simulink model "sschdlexNPCBridgeExample"  (R2023b)
settings: Solver=FixedStepDiscrete  StartTime=0.0  StopTime=0.0333  RelTol=1e-3
InitFcn:
  | ts = 1e-6;
libraries: fl_lib x17, nesl_utility x14, ee_lib x4, simulink x2, powerlib_meascontrol x2
CloseFcn:
  | clear all;
settings Model: DataTypeOverride=Off  Creator=The MathWorks, Inc.  LastModifiedBy=The MathWorks, Inc.
settings SolverCC: AlgebraicLoopSolver=TrustRegion
settings OptimizationCC: BlockReduction=off  ConditionallyExecuteInputs=off  DefaultParameterBehavior=Inlined
settings DebuggingCC: AlgebraicLoopMsg=error  SingleTaskRateTransMsg=error  UnconnectedInputMsg=warning  UnconnectedOutputMsg=warning  UnconnectedLineMsg=warning
settings HardwareCC: ProdBitPerPointer=32  ProdBitPerSizeT=32  ProdBitPerPtrDiffT=32  ProdLargestAtomicFloat=None  ProdIntDivRoundTo=Undefined  ProdEndianess=Unspecified  ProdWordSize=32  ProdHWDeviceType=ASIC/FPGA->ASIC/FPGA  TargetBitPerPointer=64  TargetBitPerSizeT=64  TargetBitPerPtrDiffT=64  TargetLongLongMode=on  TargetIntDivRoundTo=Zero  TargetEndianess=LittleEndian  TargetWordSize=64  TargetHWDeviceType=Custom Processor->MATLAB Host Computer  ProdEqTarget=off
settings ModelReferenceCC: EnableRefExpFcnMdlSchedulingChecks=on
settings RTWCC: DLArmComputeVersion=19.05

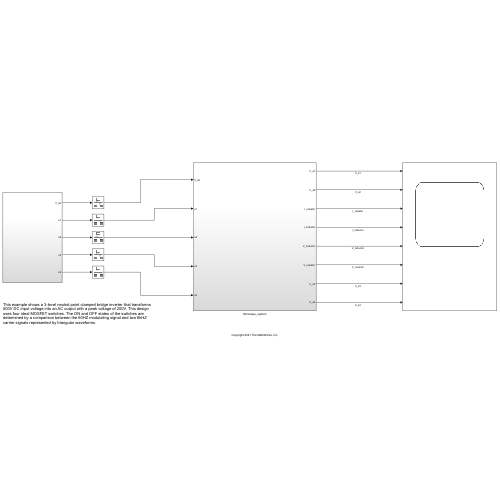
[thumbnail: Simulink's stored preview of the top-level diagram]
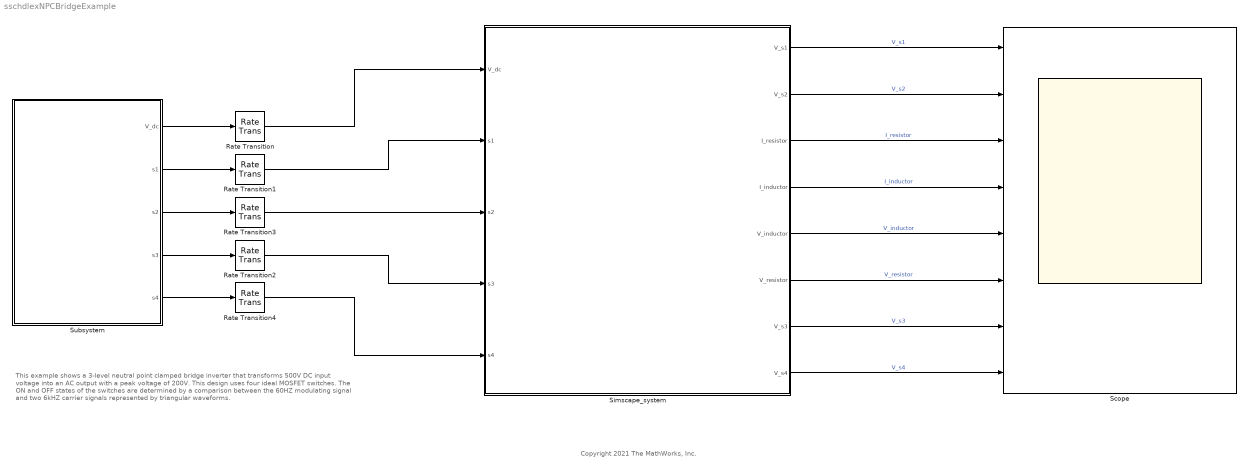
== system sschdlexNPCBridgeExample ==
  note: This example shows a 3-level neutral point clamped bridge inverter that transforms 500V DC input voltage into an AC output with a peak voltage of 200V. This design uses four ideal MOSFET switches. The ON and OFF states of the switches are determined by a comparison between the 60HZ modulating signal and two 6kHZ carrier signals represented by triangular waveforms.
  note: Copyright 2021 The MathWorks, Inc.
  Rate Transition{,1..4} (5 alike) : RateTransition
  Scope : Scope  NumInputPorts=8
  Simscape_system : Subsystem
  Subsystem : Subsystem
  wires:
  Subsystem/5(s4) -> Rate Transition4/1
  Subsystem/3(s2) -> Rate Transition3/1
  Subsystem/4(s3) -> Rate Transition2/1
  Subsystem/2(s1) -> Rate Transition1/1
  Subsystem/1(V_dc) -> Rate Transition/1
  Rate Transition/1 -> Simscape_system/1(V_dc)
  Rate Transition1/1 -> Simscape_system/2(s1)
  Rate Transition3/1 -> Simscape_system/3(s2)
  Rate Transition2/1 -> Simscape_system/4(s3)
  Rate Transition4/1 -> Simscape_system/5(s4)
  Simscape_system/1(V_s1) -> Scope/1  "V_s1"
  Simscape_system/2(V_s2) -> Scope/2  "V_s2"
  Simscape_system/3(I_resistor) -> Scope/3  "I_resistor"
  Simscape_system/4(I_inductor) -> Scope/4  "I_inductor"
  Simscape_system/5(V_inductor) -> Scope/5  "V_inductor"
  Simscape_system/6(V_resistor) -> Scope/6  "V_resistor"
  Simscape_system/7(V_s3) -> Scope/7  "V_s3"
  Simscape_system/8(V_s4) -> Scope/8  "V_s4"

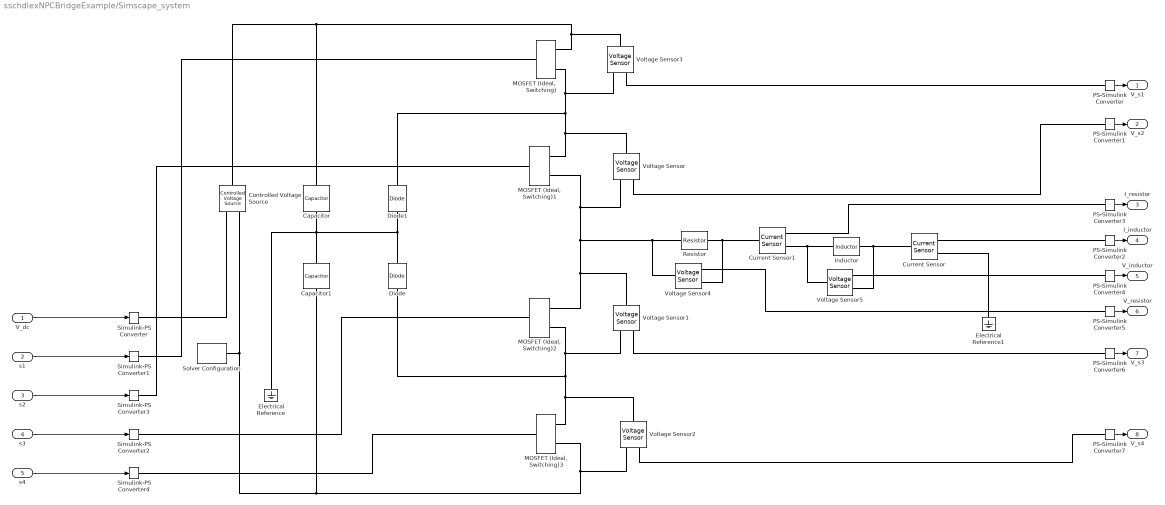
== system sschdlexNPCBridgeExample/Simscape_system ==
  V_dc : Inport
  s1 : Inport  Port=2
  s2 : Inport  Port=3
  s3 : Inport  Port=4
  s4 : Inport  Port=5
  Capacitor : fl_lib/Electrical/Electrical Elements/Capacitor  c=500e-6 F  r=0 Ohm  g=0 1/Ohm  i_specify=off  i_priority=None  i=0 A  i_nominal_specify=off  i_nominal_unit=A  i_nominal_value=1  v_specify=off  v_priority=None  v=250 V  v_nominal_specify=off  v_nominal_unit=V  v_nominal_value=1  vc_specify=on  vc_priority=High  vc=250 V  vc_nominal_specify=off  vc_nominal_unit=V  vc_nominal_value=1
  Capacitor1 : fl_lib/Electrical/Electrical Elements/Capacitor  c=500e-6 F  r=0 Ohm  g=0 1/Ohm  i_specify=off  i_priority=None  i=0 A  i_nominal_specify=off  i_nominal_unit=A  i_nominal_value=1  v_specify=off  v_priority=None  v=250 V  v_nominal_specify=off  v_nominal_unit=V  v_nominal_value=1  vc_specify=on  vc_priority=High  vc=250 V  vc_nominal_specify=off  vc_nominal_unit=V  vc_nominal_value=1
  Controlled Voltage Source : fl_lib/Electrical/Electrical Sources/Controlled Voltage Source
  Current Sensor : fl_lib/Electrical/Electrical Sensors/Current Sensor
  Current Sensor1 : fl_lib/Electrical/Electrical Sensors/Current Sensor
  Diode : fl_lib/Electrical/Electrical Elements/Diode  Vf=0.6 V  Ron=1e-3 Ohm  Goff=1e-8 1/Ohm  i_specify=off  i_priority=None  i=0 A  i_nominal_specify=off  i_nominal_unit=A  i_nominal_value=1  v_specify=off  v_priority=None  v=0 V  v_nominal_specify=off  v_nominal_unit=V  v_nominal_value=1
  Diode1 : fl_lib/Electrical/Electrical Elements/Diode  Vf=0.6 V  Ron=1e-3 Ohm  Goff=1e-8 1/Ohm  i_specify=off  i_priority=None  i=0 A  i_nominal_specify=off  i_nominal_unit=A  i_nominal_value=1  v_specify=off  v_priority=None  v=0 V  v_nominal_specify=off  v_nominal_unit=V  v_nominal_value=1
  Electrical Reference : fl_lib/Electrical/Electrical Elements/Electrical Reference
  Electrical Reference1 : fl_lib/Electrical/Electrical Elements/Electrical Reference
  Inductor : fl_lib/Electrical/Electrical Elements/Inductor  l=200e-3 H  r=0 Ohm  g=1e-9 1/Ohm  i_specify=off  i_priority=None  i=0 A  i_nominal_specify=off  i_nominal_unit=A  i_nominal_value=1  v_specify=off  v_priority=None  v=0 V  v_nominal_specify=off  v_nominal_unit=V  v_nominal_value=1  i_L_specify=off  i_L_priority=High  i_L=0 A  i_L_nominal_specify=off  i_L_nominal_unit=A  i_L_nominal_value=1
  MOSFET (Ideal, Switching){,1..3} (4 alike) : ee_lib/Semiconductors & Converters/MOSFET (Ideal, Switching)  Rds=0.001 Ohm  Goff=1e-6 1/Ohm  Vth=0.6 V  diode_param=1  diode_Vf=0.01 V  diode_Ron=0.001 Ohm  diode_Goff=1e-5 1/Ohm  diode_C=50e-9 F  diode_iRM=-235 A  diode_iF=300 A  diode_idot=-50 A/us  diode_trr_param=1  diode_trr_factor=3  diode_trr=15 us  diode_Qrr=1500 s*uA  thermal_loss_option=ee.enum.converters.thermalLossOption.constantvalues  Von_data=[0, 1.1, 1.3, 1.45, 1.75, 2.25, 2.7; 0, 1, 1.15, 1.35, 1.7, 2.35, 3] V  Eon_data=[0, .29, 1.43, 2.86, 5.71, 13.14, 22.86; 0, .57, 2.63, 5.14, 10.29, 20.57, 30.29] * 1e-3 J  Eoff_data=[0, .21, 1.07, 2.14, 4.29, 9.86, 17.14; 0, .43, 1.97, 3.86, 7.71, 15.43, 22.71] * 1e-3 J  Tj=[298.15, 398.15] K  Iout_data=[0, 10, 50, 100, 200, 400, 600] A  Eon_scalar=22.86e-3 J  Eoff_scalar=17.14e-3 J  Voff=300 V  Iout_scalar=600 A  diodeModelType=ee.enum.converters.diodeModelType.pwl  diode_IfMat=[.07, .12, .19, 1.75, 4.24, 7.32, 11.2; .16, .3, .72, 2.14, 4.02, 6.35, 9.12] A  diode_TjVec=[25, 125] degC  diode_VfVec=[.5, .7, .9, 1.3, 1.7, 2.1, 2.5] V  thermal_network_parameterization=ee.enum.thermalNetworkTopology.external  Rth=[.03, .2] K/W  Rth_Foster=[.03, .2] K/W  thermal_mass_parameterization=ee.enum.thermalNetwork.timeconstant  thermal_mass=[3, 25] J/K  thermal_mass_Foster=[33, 50] J/K  thermal_time_constant=[.1, 5] s  thermal_time_constant_Foster=[1, 10] s  thermal_mass_initial_temperatures=[25, 25] degC  junction_thermal_mass=0.1 J/K  Tau=1e-4 s  vT_specify=off  vT_priority=None  vT=0 V  vT_nominal_specify=off  vT_nominal_unit=V  vT_nominal_value=1  Qj_specify=off  Qj_priority=None  Qj=0 W  Qj_nominal_specify=off  Qj_nominal_unit=W  Qj_nominal_value=1  junction_temperature_specify=off  junction_temperature_priority=None  junction_temperature=25 degC  junction_temperature_nominal_specify=off  junction_temperature_nominal_unit=degC  junction_temperature_nominal_value=1
  PS-Simulink Converter{,1..7} (8 alike) : nesl_utility/PS-Simulink Converter  PhysicalDomain=network_engine_domain  SubClassName=ps_output  LeftPortType=input  RightPortType=output  PseudoPeriodic=off  Frequencies=[]  Unit=inherit  AffineConversion=off
  Resistor : fl_lib/Electrical/Electrical Elements/Resistor  R=100 Ohm  i_specify=off  i_priority=None  i=0 A  i_nominal_specify=off  i_nominal_unit=A  i_nominal_value=1  v_specify=off  v_priority=None  v=0 V  v_nominal_specify=off  v_nominal_unit=V  v_nominal_value=1
  Simulink-PS Converter{,1..4} (5 alike) : nesl_utility/Simulink-PS Converter  PhysicalDomain=network_engine_domain  SubClassName=ps_input  LeftPortType=input  RightPortType=output  PseudoPeriodic=off  Frequencies=[]  NoiseDistribution=none  NoiseParameters=[]  Unit=1  AffineConversion=off  FilteringAndDerivatives=provide  SimscapeFilterOrder=1  InputFilterTimeConstant=0.001  UdotUserProvided=0
  Solver Configuration : nesl_utility/Solver Configuration  PhysicalDomain=network_engine_domain  SubClassName=solver  LeftPortType=input  RightPortType=generic  Tones=[]  Harmonics=[]  SimulateNoise=off  Profile=off  UseLocalSampling=off  EnableSwitchedLinearOptims=on  FrequencyDomain=off  UseCCode=off  RelTol=0.001  AbsTol=1e-06  MinStep=1e-09  ToWorkspace=off  RevertToSquareIcSolve=off  NumHomotopyIterations=100  PhasorMode=off  PhasorModeNumHarmonics=1  DoDC=off  ResidualTolerance=1e-09  UseLocalSolver=on  LocalSolverChoice=NE_BACKWARD_EULER_ADVANCER  LocalSolverSampleTime=ts  DoFixedCost=on  MaxNonlinIter=3  MaxModeIter=2  ComputeImpulses=off  ImpulseIterations=1  LinearAlgebra=auto  EquationFormulation=NE_TIME_EF  DelaysMemoryBudget=1024  AutomaticFiltering=on  FilteringTimeConstant=0.001  PartitionStorageMethod=AS_NEEDED  PartitionMemoryBudget=1024  PartitionMethod=ROBUST
  Voltage Sensor{,1..5} (6 alike) : fl_lib/Electrical/Electrical Sensors/Voltage Sensor
  V_s1 : Outport
  V_s2 : Outport  Port=2
  I_resistor : Outport  Port=3
  I_inductor : Outport  Port=4
  V_inductor : Outport  Port=5
  V_resistor : Outport  Port=6
  V_s3 : Outport  Port=7
  V_s4 : Outport  Port=8
  wires:
  PS-Simulink Converter/1 -> V_s1/1
  s1/1 -> Simulink-PS Converter1/1
  PS-Simulink Converter7/1 -> V_s4/1
  PS-Simulink Converter6/1 -> V_s3/1
  s2/1 -> Simulink-PS Converter3/1
  s3/1 -> Simulink-PS Converter2/1
  s4/1 -> Simulink-PS Converter4/1
  PS-Simulink Converter3/1 -> I_resistor/1
  PS-Simulink Converter2/1 -> I_inductor/1
  PS-Simulink Converter4/1 -> V_inductor/1
  PS-Simulink Converter5/1 -> V_resistor/1
  V_dc/1 -> Simulink-PS Converter/1
  PS-Simulink Converter1/1 -> V_s2/1
  connections:
  PS-Simulink Converter2/LConn1 -- Current Sensor/RConn1
  Voltage Sensor1/RConn1 -- PS-Simulink Converter6/LConn1
  Simulink-PS Converter4/RConn1 -- "MOSFET (Ideal, Switching)3"/LConn1
  "MOSFET (Ideal, Switching)3"/RConn1 -- Voltage Sensor2/LConn1 -- Diode/LConn1 -- Voltage Sensor1/RConn2 -- "MOSFET (Ideal, Switching)2"/RConn2
  Voltage Sensor3/RConn1 -- PS-Simulink Converter/LConn1
  Simulink-PS Converter1/RConn1 -- "MOSFET (Ideal, Switching)"/LConn1
  Simulink-PS Converter3/RConn1 -- "MOSFET (Ideal, Switching)1"/LConn1
  Voltage Sensor/RConn1 -- PS-Simulink Converter1/LConn1
  Simulink-PS Converter2/RConn1 -- "MOSFET (Ideal, Switching)2"/LConn1
  Current Sensor1/LConn1 -- Voltage Sensor4/RConn2 -- Resistor/RConn1
  Controlled Voltage Source/LConn1 -- Voltage Sensor3/LConn1 -- "MOSFET (Ideal, Switching)"/RConn1 -- Capacitor/LConn1
  "MOSFET (Ideal, Switching)1"/RConn2 -- Voltage Sensor/RConn2 -- Voltage Sensor4/LConn1 -- Resistor/LConn1 -- Voltage Sensor1/LConn1 -- "MOSFET (Ideal, Switching)2"/RConn1
  Simulink-PS Converter/RConn1 -- Controlled Voltage Source/RConn1
  Current Sensor1/RConn2 -- Voltage Sensor5/LConn1 -- Inductor/LConn1
  "MOSFET (Ideal, Switching)3"/RConn2 -- Voltage Sensor2/RConn2 -- Controlled Voltage Source/RConn2 -- Solver Configuration/RConn1 -- Capacitor1/RConn1
  "MOSFET (Ideal, Switching)"/RConn2 -- Voltage Sensor3/RConn2 -- Diode1/RConn1 -- Voltage Sensor/LConn1 -- "MOSFET (Ideal, Switching)1"/RConn1
  Voltage Sensor5/RConn1 -- PS-Simulink Converter4/LConn1
  Voltage Sensor2/RConn1 -- PS-Simulink Converter7/LConn1
  Current Sensor1/RConn1 -- PS-Simulink Converter3/LConn1
  Voltage Sensor4/RConn1 -- PS-Simulink Converter5/LConn1
  Electrical Reference1/LConn1 -- Current Sensor/RConn2
  Inductor/RConn1 -- Voltage Sensor5/RConn2 -- Current Sensor/LConn1
  Capacitor/RConn1 -- Diode/RConn1 -- Diode1/LConn1 -- Capacitor1/LConn1 -- Electrical Reference/LConn1

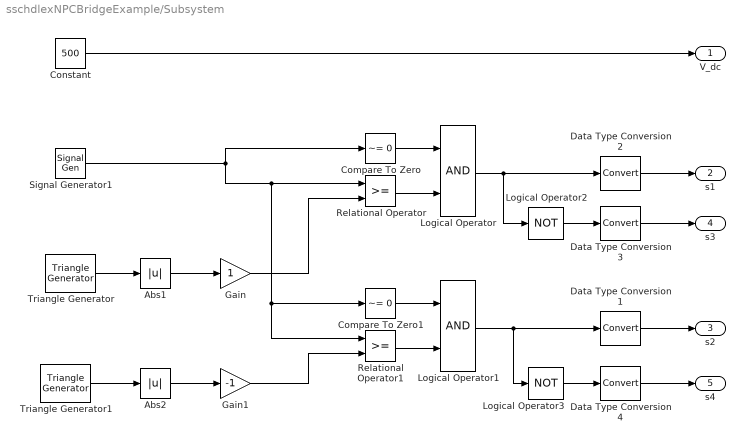
== system sschdlexNPCBridgeExample/Subsystem ==
  Abs1 : Abs  SaturateOnIntegerOverflow=off
  Abs2 : Abs  SaturateOnIntegerOverflow=off
  Compare To Zero : simulink/Logic and Bit Operations/Compare To Zero  relop=~=  OutDataTypeStr=boolean
  Compare To Zero1 : simulink/Logic and Bit Operations/Compare To Zero  relop=~=  OutDataTypeStr=boolean
  Constant : Constant  Value=500  SampleTime=-1
  Data Type Conversion{1..4} (4 alike) : DataTypeConversion  SaturateOnIntegerOverflow=off  RndMeth=Floor
  Gain : Gain
  Gain1 : Gain  Gain=-1
  Logical Operator : Logic  AllPortsSameDT=off  OutDataTypeStr=boolean
  Logical Operator1 : Logic  AllPortsSameDT=off  OutDataTypeStr=boolean
  Logical Operator2 : Logic  Operator=NOT  IconShape=distinctive  AllPortsSameDT=off  OutDataTypeStr=boolean
  Logical Operator3 : Logic  Operator=NOT  IconShape=distinctive  AllPortsSameDT=off  OutDataTypeStr=boolean
  Relational Operator : RelationalOperator  OutDataTypeStr=boolean  RndMeth=Simplest  InputSameDT=off
  Relational Operator1 : RelationalOperator  OutDataTypeStr=boolean  RndMeth=Simplest  InputSameDT=off
  Signal Generator1 : SignalGenerator  Amplitude=0.95  Frequency=60
  Triangle Generator : powerlib_meascontrol/Pulse & Signal Generators/Triangle Generator  Freq=10e3  Phase=90  Ts=0
  Triangle Generator1 : powerlib_meascontrol/Pulse & Signal Generators/Triangle Generator  Freq=10e3  Phase=0  Ts=0
  V_dc : Outport
  s1 : Outport  Port=2
  s2 : Outport  Port=3
  s3 : Outport  Port=4
  s4 : Outport  Port=5
  wires:
  Triangle Generator1/1 -> Abs2/1
  Data Type Conversion3/1 -> s3/1
  Logical Operator2/1 -> Data Type Conversion3/1
  Relational Operator/1 -> Logical Operator/2
  Constant/1 -> V_dc/1
  Logical Operator3/1 -> Data Type Conversion4/1
  Compare To Zero/1 -> Logical Operator/1
  Abs1/1 -> Gain/1
  Relational Operator1/1 -> Logical Operator1/2
  Data Type Conversion4/1 -> s4/1
  Data Type Conversion2/1 -> s1/1
  Gain/1 -> Relational Operator/2
  Signal Generator1/1 -> Compare To Zero/1, Relational Operator1/1, Compare To Zero1/1, Relational Operator/1
  Logical Operator/1 -> Data Type Conversion2/1, Logical Operator2/1
  Logical Operator1/1 -> Logical Operator3/1, Data Type Conversion1/1
  Gain1/1 -> Relational Operator1/2
  Data Type Conversion1/1 -> s2/1
  Compare To Zero1/1 -> Logical Operator1/1
  Abs2/1 -> Gain1/1
  Triangle Generator/1 -> Abs1/1
